simulink model "modell"  (R2016a)
settings: Solver=VariableStepAuto  StartTime=0.0  StopTime=10.0  RelTol=1e-3
settings Model: Creator=HaloCao  LastModifiedBy=HaloCao
settings DataIOCC: SaveFormat=Array
settings GRTTargetCC: GeneratePreprocessorConditionals=Use local settings

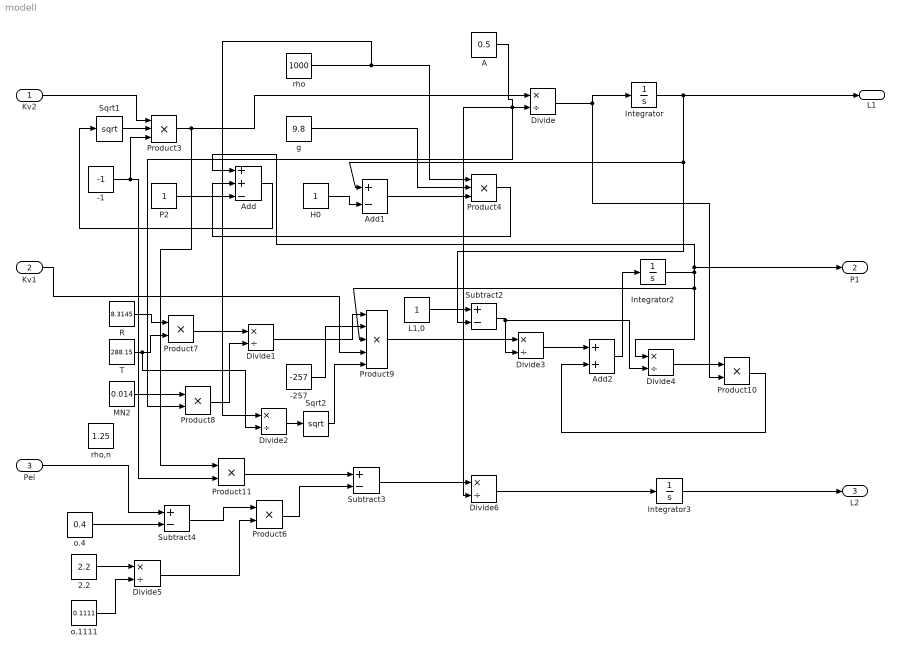
== system modell ==
  Kv2 : Inport
  Kv1 : Inport  Port=2
  Pel : Inport  Port=3
  -1 : Constant  Value=-1
  -257 : Constant  Value=-257
  2.2 : Constant  Value=2.2
  A : Constant  Value=0.5
  Add : Sum  Inputs=++-
  Add1 : Sum  Inputs=+-
  Add2 : Sum
  Divide{,1..6} (7 alike) : Product  Inputs=*/
  H0 : Constant
  Integrator : Integrator
  Integrator2 : Integrator
  Integrator3 : Integrator  InitialCondition=2
  L1,0 : Constant
  MN2 : Constant  Value=0.014
  P2 : Constant
  Product{6..8,10..11} (5 alike) : Product
  Product3 : Product  Inputs=3
  Product4 : Product  Inputs=3
  Product9 : Product  Inputs=5
  R : Constant  Value=8.3145
  Sqrt1 : Sqrt  SaturateOnIntegerOverflow=on
  Sqrt2 : Sqrt  SaturateOnIntegerOverflow=on
  Subtract2 : Sum  Inputs=+-
  Subtract3 : Sum  Inputs=+-
  Subtract4 : Sum  Inputs=+-
  T : Constant  Value=288.15
  g : Constant  Value=9.8
  o.1111 : Constant  Value=0.1111
  o.4 : Constant  Value=0.4
  rho : Constant  Value=1000
  rho,n : Constant  Value=1.25
  L1 : Outport
  P1 : Outport  Port=2
  L2 : Outport  Port=3
  wires:
  Integrator/1 -> Subtract2/2, Add1/1, L1/1
  Sqrt1/1 -> Product3/2
  Integrator3/1 -> L2/1
  Integrator2/1 -> Divide4/1, Product9/3, Add/1, P1/1
  Add/1 -> Sqrt1/1
  H0/1 -> Add1/2
  rho/1 -> Divide2/1, Product4/1
  g/1 -> Product4/2
  Add1/1 -> Product4/3
  Product4/1 -> Add/2
  P2/1 -> Add/3
  A/1 -> Divide6/2, Product8/2, Divide/2
  Divide/1 -> Integrator/1, Product10/2
  R/1 -> Product7/1
  T/1 -> Divide2/2, Product7/2
  Product7/1 -> Divide1/1
  MN2/1 -> Product8/1
  Product8/1 -> Divide1/2
  Divide1/1 -> Product9/1
  -257/1 -> Product9/2
  Divide2/1 -> Sqrt2/1
  Sqrt2/1 -> Product9/5
  Product9/1 -> Divide3/1
  L1,0/1 -> Subtract2/1
  Subtract2/1 -> Divide3/2, Divide4/2
  Divide3/1 -> Add2/1
  Divide4/1 -> Product10/1
  Product10/1 -> Add2/2
  Add2/1 -> Integrator2/1
  -1/1 -> Product11/2, Product3/3
  Product3/1 -> Product11/1, Divide/1
  Product11/1 -> Subtract3/1
  Product6/1 -> Subtract3/2
  Subtract4/1 -> Product6/1
  Divide5/1 -> Product6/2
  o.4/1 -> Subtract4/2
  2.2/1 -> Divide5/1
  o.1111/1 -> Divide5/2
  Subtract3/1 -> Divide6/1
  Divide6/1 -> Integrator3/1
  Kv1/1 -> Product9/4
  Pel/1 -> Subtract4/1
  Kv2/1 -> Product3/1
